simulink model "Clutchless_P2_Parallel"  (R2017b)
settings: Solver=FixedStepAuto  StartTime=0.0  StopTime=length(Speed)  FixedStep=0.01  MaxStep=0.01  RelTol=1e-3  EnableMultiTasking=on
PostLoadFcn:
  | , if any(exist('dsrtsu_mdlpostloadfcn', 'file') == [2, 3, 6]), try dsrtsu_mdlpostloadfcn('Execute', bdroot); catch fprintf('Error in PostLoadFcn (dsrtsu_mdlpostloadfcn) for model "%s":\n %s\n', bdroot, lasterr); end, end,
undefined symbols (not defined in the file): Actuators, APP1_OOR, APP2_OOR, APP_Mismatch, Brk_Flt, cal, Chassis, ClutchEngag, Clutchless_HSC, eng, Engine, EngineTorqueReal, EngOverTemp, ENGTRQ_MSMCH_Degraded_CP, ENGTRQ_MSMCH_ErrCritical_CP, ENGTRQ_MSMCH_LimpHome_CP, EngTrqMismatch, ess, ESSOverTemp, g, gb, Grade, KeyPos_Flt, lib_Actuators, lib_Chassis, lib_Clutchless_HSC, lib_EMachine_2017a, lib_Sensors_2017a, LossCAN, Machine, MCUOverTemp, mot, MotDirMismatch, motor_Trq, MotOverTemp, MotTrqMismatch, mph2ms, PRNDL_Flt, RegenFault, rho, Sensors, t_amb, time, tloop, veh, Vehicle
libraries: simulink x96, EC2_libraries x6, autolibmappedmotor x3, powerlib_meascontrol x2, CalculationGallon x1, lib_DCDC x1, lib_Differential x1, lib_HVESS x1, lib_Engine x1, lib_OBC x1, Scope_new x1, lib_Transmission x1
(part 2 of 10)

== system Clutchless_P2_Parallel/Camaro Plant Model/Scopes/AxlTrq_to_MtrTrq2 ==
  note: //From motor axle torque to motor torque//
  In1 : Inport
  Compare To Constant : simulink/Logic and Bit Operations/Compare To Constant  relop===  const=0  OutDataTypeStr=boolean
  Constant1 : Constant  Value=max(gb.plant.init.ratio.map)
  Constant5 : Constant  Value=fd.plant.init.ratio
  Divide : Product  Inputs=*//
  Rate Limiter : RateLimiter  RisingSlewLimit=mcu.plant.init.trq_uprate  FallingSlewLimit=mcu.plant.init.trq_derate
  Ratio Filter : Subsystem
  Switch : Switch  Criteria=u2 > Threshold
  Out1 : Outport
  wires:
  In1/1 -> Divide/1
  Constant5/1 -> Divide/2
  Divide/1 -> Rate Limiter/1
  [TransRatio] -> Ratio Filter/1(Ratio)
  Compare To Constant/1 -> Switch/2
  Constant1/1 -> Switch/1
  Rate Limiter/1 -> Out1/1
  Switch/1 -> Divide/3
  Ratio Filter/1(Filtered_Ratio) -> Switch/3, Compare To Constant/1

== system Clutchless_P2_Parallel/Clutchless_HSC/HSC/Camaro Fault Detection ==
  Sensors : Inport
  Component Diagnostic : Subsystem
  Input Conversions : Subsystem
  Signal Diagnostic : Subsystem
  SystemDiag : lib_SystemDiag/SystemDiag
  Diagnostic : Outport
  wires:
  Signal Diagnostic/1(SignalDiag) -> Component Diagnostic/1(SignalDiag)
  Component Diagnostic/1(CompDiag) -> SystemDiag/1
  Input Conversions/1(VehSig) -> Signal Diagnostic/1(VehSig)
  Sensors/1 -> Input Conversions/1(RawSig)
  SystemDiag/1 -> Diagnostic/1

== system Clutchless_P2_Parallel/Clutchless_HSC/HSC/Driver_Requests ==
  note: Driver management
  Sensors : Inport
  "Diagnostic " : Inport  Port=2
  "Controls " : Inport  Port=3
  APP_BPP to DrvIntndAxlTrq2 : Subsystem
  DriverRequests : Outport
  wires:
  "Controls "/1 -> APP_BPP to DrvIntndAxlTrq2/3(Controls)
  "Diagnostic "/1 -> APP_BPP to DrvIntndAxlTrq2/2(Diag)
  APP_BPP to DrvIntndAxlTrq2/1(IntndAxlTrq) -> DriverRequests/1
  Sensors/1 -> APP_BPP to DrvIntndAxlTrq2/1(Sensors)

== system Clutchless_P2_Parallel/Clutchless_HSC/HSC/Powertrain Manager ==
  Sensors : Inport
  Driver Request : Inport  Port=2
  Fault Detection : Inport  Port=3
  Ground : Ground
  HV Manager : Subsystem  AncestorBlock=lib_HVManager_PostIMG_2017a/HV Manager
  Output Conversion : Subsystem
  Thermal Manager : Subsystem  AncestorBlock=lib_ThermalManager/Thermal Manager
  Torque Distribution : Subsystem  AncestorBlock=lib_TorqueDistribution_2017a/Torque Distribution
  Out1 : Outport
  Controls : Outport  Port=2
  tag scope: HV_BUS_Status=global
  wires:
  Torque Distribution/1(Controls) -> HV Manager/2(Controls), Controls/1, [Controls]
  Ground/1 -> Output Conversion/9(In11)  "Trans_test"
  HV Manager/1(BMS_CAN) -> [BMS_CAN]
  HV Manager/2(HV_BUS_Status) -> [HV_BUS_Status]
  HV Manager/4(OBC_Digital) -> [OBC_Digital]
  HV Manager/3(OBC_CAN) -> [OBC_CAN]
  Driver Request/1 -> Torque Distribution/2(Driver Request)
  [BMS_CAN] -> Output Conversion/1(In1)  "BMS_CAN"
  [OBC_CAN] -> Output Conversion/2(In2)  "OBC_CAN"
  [MCU_CAN] -> Output Conversion/3(In3)  "MCU_CAN"
  [Controls] -> Output Conversion/4(In4)  "Controls"
  Output Conversion/1(Out1) -> Out1/1
  HV Manager/5(BMS_Digital) -> [BMS_Digital]
  [BMS_Digital] -> Output Conversion/5(In5)  "BMS_Digital"
  Fault Detection/1 -> Torque Distribution/3(Fault Detection)
  Thermal Manager/1(Out1) -> [Fuel_Pump_Control]
  HV Manager/6(Axiomatic_CAN) -> [Axiomatic_CAN]
  [Axiomatic_CAN] -> Output Conversion/8(In10)  "Axiomatic_CAN"
  [OBC_Digital] -> Output Conversion/7(In9)  "OBC_Digital"
  [Fuel_Pump_Control] -> Output Conversion/6(In8)  "Fuel_Pump_Control"
  Sensors/1 -> Thermal Manager/1(In2), HV Manager/1(Sensors), Torque Distribution/1(Sensors)

== system Clutchless_P2_Parallel/Fault Trigger /Component Diagnostics setting/Mismch type ==
  In1 : Inport
  Constant : Constant  Value=cal.ENGTRQ_MSMCH.Degraded_CP+1
  Constant1 : Constant  Value=cal.ENGTRQ_MSMCH.LimpHome_CP+1
  Constant2 : Constant  Value=cal.ENGTRQ_MSMCH.ErrCritical_CP+1
  Constant3 : Constant  Value=0
  Multiport Switch : MultiPortSwitch  DataPortOrder=Zero-based contiguous  Inputs=4
  Out1 : Outport
  wires:
  Constant1/1 -> Multiport Switch/4
  Constant2/1 -> Multiport Switch/5
  In1/1 -> Multiport Switch/1
  Multiport Switch/1 -> Out1/1
  Constant3/1 -> Multiport Switch/2
  Constant/1 -> Multiport Switch/3

== system Clutchless_P2_Parallel/Fault Trigger /Component Diagnostics setting/Mismch type1 ==
  In1 : Inport
  Constant : Constant  Value=cal.MOTTRQ_MSMCH.Degraded_CP+1
  Constant1 : Constant  Value=cal.MOTTRQ_MSMCH.LimpHome_CP+1
  Constant2 : Constant  Value=cal.ENGTRQ_MSMCH.ErrCritical_CP+1
  Constant3 : Constant  Value=0
  Multiport Switch : MultiPortSwitch  DataPortOrder=Zero-based contiguous  Inputs=4
  Out1 : Outport
  wires:
  Constant/1 -> Multiport Switch/3
  Constant3/1 -> Multiport Switch/2
  Multiport Switch/1 -> Out1/1
  In1/1 -> Multiport Switch/1
  Constant2/1 -> Multiport Switch/5
  Constant1/1 -> Multiport Switch/4

== system Clutchless_P2_Parallel/Fault Trigger /Component Diagnostics setting/Override  ClutchEngag ==
  note: Override Switch Subsystem
  note: This subsystem is used to override the model value of a signal to a constant value
  In1 : Inport
  Constant : Constant  Value=0
  Multiport Switch : MultiPortSwitch  DataPortOrder=Zero-based contiguous  Inputs=2
  Signal Override Switch 0 = Use Model 1 = Use Constant : Constant  Value=ClutchEngagFlt
  Out1 : Outport
  wires:
  Constant/1 -> Multiport Switch/3
  Multiport Switch/1 -> Out1/1
  In1/1 -> Multiport Switch/2
  Signal Override Switch 0 = Use Model 1 = Use Constant/1 -> Multiport Switch/1

== system Clutchless_P2_Parallel/Fault Trigger /Component Diagnostics setting/Override  ESSOverTemp ==
  note: This subsystem is used to override the model value of a signal to a constant value
  note: Override Switch Subsystem
  In1 : Inport
  Constant : Constant  Value=0
  Multiport Switch : MultiPortSwitch  DataPortOrder=Zero-based contiguous  Inputs=2
  Signal Override Switch 0 = Use Model 1 = Use Constant : Constant  Value=ESSOverTemp_ON
  Out1 : Outport
  wires:
  Signal Override Switch 0 = Use Model 1 = Use Constant/1 -> Multiport Switch/1
  In1/1 -> Multiport Switch/2
  Multiport Switch/1 -> Out1/1
  Constant/1 -> Multiport Switch/3

== system Clutchless_P2_Parallel/Fault Trigger /Component Diagnostics setting/Override  EngOverTemp ==
  note: Override Switch Subsystem
  note: This subsystem is used to override the model value of a signal to a constant value
  In1 : Inport
  Constant : Constant  Value=0
  Multiport Switch : MultiPortSwitch  DataPortOrder=Zero-based contiguous  Inputs=2
  Signal Override Switch 0 = Use Model 1 = Use Constant : Constant  Value=EngOverTemp_ON
  Out1 : Outport
  wires:
  Constant/1 -> Multiport Switch/3
  Multiport Switch/1 -> Out1/1
  In1/1 -> Multiport Switch/2
  Signal Override Switch 0 = Use Model 1 = Use Constant/1 -> Multiport Switch/1

== system Clutchless_P2_Parallel/Fault Trigger /Component Diagnostics setting/Override  EngTrqMismatch ==
  note: This subsystem is used to override the model value of a signal to a constant value
  note: Override Switch Subsystem
  In1 : Inport
  Constant : Constant  Value=0
  Multiport Switch : MultiPortSwitch  DataPortOrder=Zero-based contiguous  Inputs=2
  Signal Override Switch 0 = Use Model 1 = Use Constant : Constant  Value=EngTrqMismatch_ON
  Out1 : Outport
  wires:
  Signal Override Switch 0 = Use Model 1 = Use Constant/1 -> Multiport Switch/1
  In1/1 -> Multiport Switch/2
  Multiport Switch/1 -> Out1/1
  Constant/1 -> Multiport Switch/3

== system Clutchless_P2_Parallel/Fault Trigger /Component Diagnostics setting/Override  LossCAN ==
  note: Override Switch Subsystem
  note: This subsystem is used to override the model value of a signal to a constant value
  In1 : Inport
  Constant : Constant  Value=0
  Multiport Switch : MultiPortSwitch  DataPortOrder=Zero-based contiguous  Inputs=2
  Signal Override Switch 0 = Use Model 1 = Use Constant : Constant  Value=LossCAN_ON
  Out1 : Outport
  wires:
  Constant/1 -> Multiport Switch/3
  Multiport Switch/1 -> Out1/1
  In1/1 -> Multiport Switch/2
  Signal Override Switch 0 = Use Model 1 = Use Constant/1 -> Multiport Switch/1

== system Clutchless_P2_Parallel/Fault Trigger /Component Diagnostics setting/Override  MCUOverTemp ==
  note: This subsystem is used to override the model value of a signal to a constant value
  note: Override Switch Subsystem
  In1 : Inport
  Constant : Constant  Value=0
  Multiport Switch : MultiPortSwitch  DataPortOrder=Zero-based contiguous  Inputs=2
  Signal Override Switch 0 = Use Model 1 = Use Constant : Constant  Value=MCUOverTemp_ON
  Out1 : Outport
  wires:
  Signal Override Switch 0 = Use Model 1 = Use Constant/1 -> Multiport Switch/1
  In1/1 -> Multiport Switch/2
  Multiport Switch/1 -> Out1/1
  Constant/1 -> Multiport Switch/3

== system Clutchless_P2_Parallel/Fault Trigger /Component Diagnostics setting/Override  MotDirMismatch ==
  note: Override Switch Subsystem
  note: This subsystem is used to override the model value of a signal to a constant value
  In1 : Inport
  Constant : Constant  Value=0
  Multiport Switch : MultiPortSwitch  DataPortOrder=Zero-based contiguous  Inputs=2
  Signal Override Switch 0 = Use Model 1 = Use Constant : Constant  Value=MotDirMismatch_ON
  Out1 : Outport
  wires:
  Constant/1 -> Multiport Switch/3
  Multiport Switch/1 -> Out1/1
  In1/1 -> Multiport Switch/2
  Signal Override Switch 0 = Use Model 1 = Use Constant/1 -> Multiport Switch/1

== system Clutchless_P2_Parallel/Fault Trigger /Component Diagnostics setting/Override  MotOverTemp ==
  note: Override Switch Subsystem
  note: This subsystem is used to override the model value of a signal to a constant value
  In1 : Inport
  Constant : Constant  Value=0
  Multiport Switch : MultiPortSwitch  DataPortOrder=Zero-based contiguous  Inputs=2
  Signal Override Switch 0 = Use Model 1 = Use Constant : Constant  Value=MotOverTemp_ON
  Out1 : Outport
  wires:
  Constant/1 -> Multiport Switch/3
  Multiport Switch/1 -> Out1/1
  In1/1 -> Multiport Switch/2
  Signal Override Switch 0 = Use Model 1 = Use Constant/1 -> Multiport Switch/1

== system Clutchless_P2_Parallel/Fault Trigger /Component Diagnostics setting/Override  MotTrqMismatch ==
  note: This subsystem is used to override the model value of a signal to a constant value
  note: Override Switch Subsystem
  In1 : Inport
  Constant : Constant  Value=0
  Multiport Switch : MultiPortSwitch  DataPortOrder=Zero-based contiguous  Inputs=2
  Signal Override Switch 0 = Use Model 1 = Use Constant : Constant  Value=MotTrqMismatch_ON
  Out1 : Outport
  wires:
  Signal Override Switch 0 = Use Model 1 = Use Constant/1 -> Multiport Switch/1
  In1/1 -> Multiport Switch/2
  Multiport Switch/1 -> Out1/1
  Constant/1 -> Multiport Switch/3

== system Clutchless_P2_Parallel/Fault Trigger /Driver Interface Diagnostics setting/Override  APP1_OOR ==
  note: Signal Override Switch
      | 0 = Use Model
      | 1 = Use Constant
  note: Override Switch Subsystem
  note: This subsystem is used to override the model value of a signal to a constant value
  In1 : Inport
  APP1_OOR_ON : Constant  Value=APP1_OOR_ON
  Constant : Constant  Value=0
  Multiport Switch : MultiPortSwitch  DataPortOrder=Zero-based contiguous  Inputs=2
  Out1 : Outport
  wires:
  Constant/1 -> Multiport Switch/3
  Multiport Switch/1 -> Out1/1
  In1/1 -> Multiport Switch/2
  APP1_OOR_ON/1 -> Multiport Switch/1

== system Clutchless_P2_Parallel/Fault Trigger /Driver Interface Diagnostics setting/Override  APP2_OOR ==
  note: Signal Override Switch
      | 0 = Use Model
      | 1 = Use Constant
  note: This subsystem is used to override the model value of a signal to a constant value
  note: Override Switch Subsystem
  In1 : Inport
  APP2_OOR_ON : Constant  Value=APP2_OOR_ON
  Constant : Constant  Value=0
  Multiport Switch : MultiPortSwitch  DataPortOrder=Zero-based contiguous  Inputs=2
  Out1 : Outport
  wires:
  APP2_OOR_ON/1 -> Multiport Switch/1
  In1/1 -> Multiport Switch/2
  Multiport Switch/1 -> Out1/1
  Constant/1 -> Multiport Switch/3

== system Clutchless_P2_Parallel/Fault Trigger /Driver Interface Diagnostics setting/Override  APP_Mismatch ==
  note: Signal Override Switch
      | 0 = Use Model
      | 1 = Use Constant
  note: Override Switch Subsystem
  note: This subsystem is used to override the model value of a signal to a constant value
  In1 : Inport
  APP_Mismatch_Override : Constant  Value=Mismatch_APP_ON
  Constant : Constant  Value=0
  Multiport Switch : MultiPortSwitch  DataPortOrder=Zero-based contiguous  Inputs=2
  Out1 : Outport
  wires:
  Constant/1 -> Multiport Switch/3
  Multiport Switch/1 -> Out1/1
  In1/1 -> Multiport Switch/2
  APP_Mismatch_Override/1 -> Multiport Switch/1

== system Clutchless_P2_Parallel/Fault Trigger /Driver Interface Diagnostics setting/Override  BPP_Flt ==
  note: Signal Override Switch
      | 0 = Use Model
      | 1 = Use Constant
  note: This subsystem is used to override the model value of a signal to a constant value
  note: Override Switch Subsystem
  In1 : Inport
  Brk_Flt_ON : Constant  Value=Brk_Flt_ON
  Constant : Constant  Value=0
  Multiport Switch : MultiPortSwitch  DataPortOrder=Zero-based contiguous  Inputs=2
  Out1 : Outport
  wires:
  Brk_Flt_ON/1 -> Multiport Switch/1
  In1/1 -> Multiport Switch/2
  Multiport Switch/1 -> Out1/1
  Constant/1 -> Multiport Switch/3

== system Clutchless_P2_Parallel/Fault Trigger /Driver Interface Diagnostics setting/Override  KeyPos_Flt ==
  note: Signal Override Switch
      | 0 = Use Model
      | 1 = Use Constant
  note: Override Switch Subsystem
  note: This subsystem is used to override the model value of a signal to a constant value
  In1 : Inport
  Constant : Constant  Value=0
  KeyPos_Flt_ON : Constant  Value=KeyPos_Flt_ON
  Multiport Switch : MultiPortSwitch  DataPortOrder=Zero-based contiguous  Inputs=2
  Out1 : Outport
  wires:
  Constant/1 -> Multiport Switch/3
  Multiport Switch/1 -> Out1/1
  In1/1 -> Multiport Switch/2
  KeyPos_Flt_ON/1 -> Multiport Switch/1

== system Clutchless_P2_Parallel/Fault Trigger /Driver Interface Diagnostics setting/Override  PRNDL_Flt ==
  note: Signal Override Switch
      | 0 = Use Model
      | 1 = Use Constant
  note: This subsystem is used to override the model value of a signal to a constant value
  note: Override Switch Subsystem
  In1 : Inport
  Constant : Constant  Value=0
  Multiport Switch : MultiPortSwitch  DataPortOrder=Zero-based contiguous  Inputs=2
  PRNDL_Flt_ON : Constant  Value=PRNDL_Flt_ON
  Out1 : Outport
  wires:
  PRNDL_Flt_ON/1 -> Multiport Switch/1
  In1/1 -> Multiport Switch/2
  Multiport Switch/1 -> Out1/1
  Constant/1 -> Multiport Switch/3

== system Clutchless_P2_Parallel/Sensors/CAN/EBCAN ==
  In1 : Inport
  BMS_Antrieb : Subsystem
  Bus Creator : BusCreator  Inputs=3
  Bus Selector : BusSelector  OutputSignals=ECM_CAN,BMS_CAN.BMS_Hybrid
  CCM : Subsystem
  ECM : Subsystem
  Out1 : Outport
  wires:
  Bus Selector/2 -> CCM/1(In1), BMS_Antrieb/1(In1)  "<BMS_Hybrid>"
  Bus Selector/1 -> ECM/1(In1)  "<ECM_CAN>"
  In1/1 -> Bus Selector/1
  CCM/1(Out1) -> Bus Creator/3  "from_CCM"
  Bus Creator/1 -> Out1/1
  BMS_Antrieb/1(Out1) -> Bus Creator/2  "from_BMSAntrieb"
  ECM/1(Out1) -> Bus Creator/1  "from_ECM"

== system Clutchless_P2_Parallel/Sensors/CAN/HV_CAN ==
  In1 : Inport
  BMS_Hybrid : Subsystem
  Bus Creator : BusCreator  Inputs=3
  Bus Selector : BusSelector  OutputSignals=MCU_CAN,BMS_CAN.BMS_Plugin,OBC_CAN
  MCU : Subsystem
  OBC : Subsystem
  Out1 : Outport
  wires:
  Bus Selector/3 -> OBC/1(In1)  "<OBC_CAN>"
  Bus Selector/2 -> BMS_Hybrid/1(In1)  "<BMS_Plugin>"
  Bus Selector/1 -> MCU/1(In1)  "<MCU_CAN>"
  In1/1 -> Bus Selector/1
  Bus Creator/1 -> Out1/1
  OBC/1(Out1) -> Bus Creator/3  "from_OBC"
  BMS_Hybrid/1(Out1) -> Bus Creator/2  "from_BMSHybrid"
  MCU/1(Out1) -> Bus Creator/1  "from_MCU"

== system Clutchless_P2_Parallel/Sensors/CAN/VEH_CAN ==
  In1 : Inport
  BCM : Subsystem
  Bus Creator : BusCreator  Inputs=4
  Bus Selector : BusSelector  OutputSignals=TCM_CAN,BCM_CAN
  EBCM : Subsystem  Commented=on
  Ground : Ground  Commented=on
  Ground1 : Ground  Commented=on
  ICCM : Subsystem  Commented=on
  TCM : Subsystem
  Out1 : Outport
  wires:
  Ground/1 -> EBCM/1(In1)  "<EBCM>"
  Ground1/1 -> ICCM/1(In1)  "<ONSTAR>"
  Bus Selector/2 -> BCM/1(In1)  "<BCM_CAN>"
  Bus Selector/1 -> TCM/1(In1)  "<TCM_CAN>"
  Bus Creator/1 -> Out1/1
  EBCM/1(Out1) -> Bus Creator/4  "from_EBCM"
  ICCM/1(Out1) -> Bus Creator/3  "from_ICCM"
  BCM/1(Out1) -> Bus Creator/2  "from_BCM"
  TCM/1(Out1) -> Bus Creator/1  "from_TCM"
  In1/1 -> Bus Selector/1

== system Clutchless_P2_Parallel/Actuators/CAN/EBCAN/ISO_Hybrid_01_Req ==
  In1 : Inport
  Bus Creator : BusCreator  Inputs=1
  Bus Selector : BusSelector  OutputSignals=ISO_Hybrid_01_Req_Data_byte_3
  Data Type Conversion : DataTypeConversion
  Out1 : Outport
  wires:
  In1/1 -> Bus Selector/1
  Data Type Conversion/1 -> Bus Creator/1  "ISO_Hybrid_01_Req_Data_4"
  Bus Creator/1 -> Out1/1  "ISO_Hybrid_01_Req"
  Bus Selector/1 -> Data Type Conversion/1  "<ISO_Hybrid_01_Req_Data_byte_3>"

== system Clutchless_P2_Parallel/Actuators/CAN/EBCAN/PPEI_Platform_General_Status ==
  In1 : Inport
  Bus Creator : BusCreator  Inputs=1
  Data Type Conversion : DataTypeConversion
  Out1 : Outport
  wires:
  Bus Creator/1 -> Out1/1  "PPEI_Platform_General_Status"
  Data Type Conversion/1 -> Bus Creator/1  "SysPwrMd"
  In1/1 -> Data Type Conversion/1

== system Clutchless_P2_Parallel/Actuators/CAN/EBCAN/PPEI_Trans_General_Status_2 ==
  In1 : Inport
  Bus Creator : BusCreator  Inputs=1
  Data Type Conversion : DataTypeConversion
  Out1 : Outport
  wires:
  In1/1 -> Data Type Conversion/1
  Data Type Conversion/1 -> Bus Creator/1  "TrnsShftLvrPos"
  Bus Creator/1 -> Out1/1  "PPEI_Trans_General_Status_2"

== system Clutchless_P2_Parallel/Actuators/CAN/VEH_CAN/BCM ==
  In1 : Inport
  Bus Creator : BusCreator  Inputs=1
  Bus Selector : BusSelector  OutputSignals=Controls.powerMode
  Out1 : Outport
  wires:
  In1/1 -> Bus Selector/1
  Bus Selector/1 -> Bus Creator/1  "<powerMode>"
  Bus Creator/1 -> Out1/1

== system Clutchless_P2_Parallel/Actuators/CAN/VEH_CAN/EBCM ==
  In1 : Inport
  Out1 : Outport
  wires:
  In1/1 -> Out1/1

== system Clutchless_P2_Parallel/Actuators/CAN/VEH_CAN/ICCM ==
  In1 : Inport
  Out1 : Outport
  wires:
  In1/1 -> Out1/1

== system Clutchless_P2_Parallel/Camaro Plant Model/E-Machine/IMG Plant/ Actuators ==
  In1 : Inport
  Bus Selector : BusSelector  OutputSignals=MotTrqCmd,Direction_Command,InverterEnabled
  MotTrqCmd : Outport
  DirectionCommand : Outport  Port=2
  InverterEnabled : Outport  Port=3
  wires:
  In1/1 -> Bus Selector/1
  Bus Selector/1 -> MotTrqCmd/1  "<MotTrqCmd>"
  Bus Selector/2 -> DirectionCommand/1  "<Direction_Command>"
  Bus Selector/3 -> InverterEnabled/1  "<InverterEnabled>"

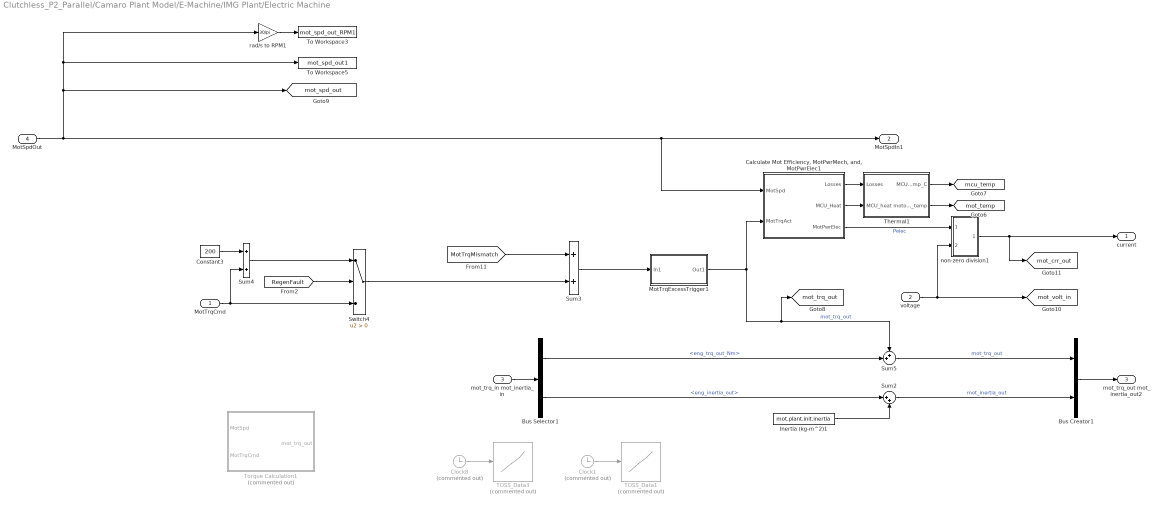
== system Clutchless_P2_Parallel/Camaro Plant Model/E-Machine/IMG Plant/Electric Machine ==
  MotTrqCmd : Inport
  voltage : Inport  Port=2
  mot_trq_in mot_inertia_in : Inport  Port=3
  MotSpdOut : Inport  Port=4
  Bus Creator1 : BusCreator  Inputs=2
  Bus Selector1 : BusSelector  OutputSignals=eng_trq_out_Nm,eng_inertia_out
  "Calculate Mot Efficiency, MotPwrMech, and, MotPwrElec1" : Subsystem
  Clock1 : Clock  Commented=on
  Clock8 : Clock  Commented=on
  Constant3 : Constant  Value=200
  Inertia (kg-m^2)1 : Constant  Value=mot.plant.init.inertia
  MotTrqExcessTrigger1 : Subsystem
  Sum2 : Sum  Inputs=|++
  Sum3 : Sum
  Sum4 : Sum
  Sum5 : Sum  Inputs=++|
  Switch4 : Switch  Criteria=u2 > Threshold
  TOSS_Data1 : Lookup_n-D  Commented=on  NumberOfTableDimensions=1  BreakpointsForDimension1=time  Table=EngineTorqueReal  InternalRulePriority=Speed  RndMeth=Simplest  InputSameDT=on
  TOSS_Data3 : Lookup_n-D  Commented=on  NumberOfTableDimensions=1  BreakpointsForDimension1=time  Table=motor_Trq  InternalRulePriority=Speed  RndMeth=Simplest  InputSameDT=on
  Thermal1 : Subsystem
  To Workspace3 : ToWorkspace  VariableName=mot_spd_out_RPM1  SampleTime=-1
      settings: Decimation=WORKSPACE_DECIMATION
  To Workspace5 : ToWorkspace  VariableName=mot_spd_out1  SampleTime=-1
      settings: Decimation=WORKSPACE_DECIMATION
  Torque Calculation1 : Subsystem  Commented=on
  non-zero division1 : Subsystem
      mask Display: disp('divider \n I1/I2')
  rad/s to RPM1 : Gain  Gain=30/pi
  current : Outport
  MotSpdIn1 : Outport  Port=2
  mot_trq_out mot_inertia_out2 : Outport  Port=3
  tag scope: mcu_temp=global, mot_crr_out=global, mot_spd_out=global, mot_temp=global, mot_trq_out=global, mot_volt_in=global
  wires:
  Thermal1/1(MCU_temp_C) -> [mcu_temp]
  Thermal1/2(motor_temp) -> [mot_temp]
  Constant3/1 -> Sum4/1
  [RegenFault] -> Switch4/2
  "Calculate Mot Efficiency, MotPwrMech, and, MotPwrElec1"/1(Losses) -> Thermal1/1(Losses)
  Sum4/1 -> Switch4/1
  Sum3/1 -> MotTrqExcessTrigger1/1(In1)
  "Calculate Mot Efficiency, MotPwrMech, and, MotPwrElec1"/2(MCU_Heat) -> Thermal1/2(MCU_heat)
  Switch4/1 -> Sum3/2
  "Calculate Mot Efficiency, MotPwrMech, and, MotPwrElec1"/3(MotPwrElec) -> non-zero division1/1(In1)  "Pelec"
  non-zero division1/1(Out1) -> [mot_crr_out], current/1
  MotTrqExcessTrigger1/1(Out1) -> [mot_trq_out], Sum5/1, "Calculate Mot Efficiency, MotPwrMech, and, MotPwrElec1"/2(MotTrqAct)  "mot_trq_out"
  MotTrqCmd/1 -> Sum4/2, Switch4/3
  voltage/1 -> non-zero division1/2(In2), [mot_volt_in]
  [MotTrqMismatch] -> Sum3/1
  Sum5/1 -> Bus Creator1/1  "mot_trq_out"
  Inertia (kg-m^2)1/1 -> Sum2/2
  Sum2/1 -> Bus Creator1/2  "mot_inertia_out"
  Bus Creator1/1 -> mot_trq_out mot_inertia_out2/1
  mot_trq_in mot_inertia_in/1 -> Bus Selector1/1
  Bus Selector1/2 -> Sum2/1  "<eng_inertia_out>"
  Bus Selector1/1 -> Sum5/2  "<eng_trq_out_Nm>"
  rad/s to RPM1/1 -> To Workspace3/1
  MotSpdOut/1 -> "Calculate Mot Efficiency, MotPwrMech, and, MotPwrElec1"/1(MotSpd), MotSpdIn1/1, [mot_spd_out], To Workspace5/1, rad/s to RPM1/1
  Clock8/1 -> TOSS_Data3/1
  Clock1/1 -> TOSS_Data1/1

== system Clutchless_P2_Parallel/Camaro Plant Model/E-Machine/IMG Plant/Sensors ==
  In2 : Inport
  In3 : Inport  Port=2
  In4 : Inport  Port=3
  In5 : Inport  Port=4
  In6 : Inport  Port=5
  In1 : Inport  Port=6
  In7 : Inport  Port=7
  Bus Creator : BusCreator  Inputs=7
  Out1 : Outport
  wires:
  Bus Creator/1 -> Out1/1
  In2/1 -> Bus Creator/1  "mot_spd_out"
  In4/1 -> Bus Creator/3  "mot_crr_out"
  In5/1 -> Bus Creator/4  "mot_volt_in"
  In3/1 -> Bus Creator/2  "mot_trq_out"
  In6/1 -> Bus Creator/5  "mot_temp"
  In1/1 -> Bus Creator/6  "mcu_temp"
  In7/1 -> Bus Creator/7  "clt_plant_spd_in"

== system Clutchless_P2_Parallel/Camaro Plant Model/E-Machine/IMG Plant2/ Actuators ==
  In1 : Inport
  Bus Selector : BusSelector  OutputSignals=MotTrqCmd,Direction_Command,InverterEnabled
  Out2 : Outport
  Out3 : Outport  Port=2
  Out4 : Outport  Port=3
  wires:
  Bus Selector/3 -> Out4/1  "<InverterEnabled>"
  Bus Selector/2 -> Out3/1  "<Direction_Command>"
  In1/1 -> Bus Selector/1
  Bus Selector/1 -> Out2/1  "<MotTrqCmd>"

== system Clutchless_P2_Parallel/Camaro Plant Model/E-Machine/IMG Plant2/Calculate Mot Efficiency, MotPwrMech, and, MotPwrElec ==
  note: Pelec_req = Pmech_req*Eff^k,
      | k = -1 if Trq >= 0,
      | k = 1 if Trq < 0
  MotSpd : Inport
  MotTrqAct : Inport  Port=2
  -1 : Gain  Gain=8
  "-1 when + 1 when - " : Gain  Gain=-1
  -2 : Gain  Gain=tloop
  2-D Lookup Table : Lookup_n-D  BreakpointsForDimension1=mot.plant.init.eff_trq.idx2_trq  BreakpointsForDimension2=mot.plant.init.eff_trq.idx1_spd  Table=mot.plant.init.eff_trq.map  InternalRulePriority=Speed  RndMeth=Simplest  InputSameDT=on
  Abs{,1..3} (4 alike) : Abs
  Add : Sum  Inputs=-+
  Add1 : Sum  Inputs=+-
  Add2 : Sum  Commented=on
  Constant : Constant  Value=1-0.8
  Constant1 : Constant  Commented=on  Value=mot.plant.init.mcu_mass
  Constant2 : Constant  Commented=on  Value=mot.plant.init.specific_heat
  Divide : Product  Commented=on  Inputs=*/
  Gain2 : Gain  Gain=1/100
  Lower Limit : Subsystem  Commented=on  mask{Lolimit=t_amb+20}
      mask prompts: Lolimit "Lower Limit"
  MCUOverTemp Fault : Subsystem  Commented=on
  MCU_WEGPmp : Constant  Value=0
  Math Function1 : Math  Operator=pow  SaturateOnIntegerOverflow=on
  Memory : Memory
  Memory1 : Memory  Commented=on
  Product : Product
  Product1 : Product
  Product2 : Product
  Product3 : Product  Commented=on
  Sign : Signum
  rad/s to rpm : Gain  Gain=30/pi
  Losses : Outport
  MotPwrElec : Outport  Port=2
  MCU_Heat : Outport  Port=3
  wires:
  Lower Limit/1(Out1) -> Memory1/1, MCUOverTemp Fault/1(In1)
  Add2/1 -> Lower Limit/1(In1)
  Memory1/1 -> Add2/2
  Divide/1 -> Add2/1
  Product3/1 -> Divide/2
  Constant2/1 -> Product3/2
  Constant1/1 -> Product3/1
  -2/1 -> MCU_Heat/1
  -1/1 -> Add1/2
  Add1/1 -> -2/1
  MCU_WEGPmp/1 -> -1/1
  Abs3/1 -> Add1/1
  Product2/1 -> Abs3/1
  Constant/1 -> Product2/2
  Memory/1 -> Sign/1
  Math Function1/1 -> Product1/2
  Add/1 -> Abs2/1
  Abs2/1 -> Losses/1
  "-1 when + 1 when - "/1 -> Math Function1/2
  MotSpd/1 -> rad/s to rpm/1, Product/2
  MotTrqAct/1 -> Abs/1, Product/1, Memory/1
  Product/1 -> Product1/1, Add/1  "MotPwrMech"
  Product1/1 -> MotPwrElec/1, Add/2, Product2/1  "MotPwrElec"
  2-D Lookup Table/1 -> Gain2/1
  Gain2/1 -> Math Function1/1
  Abs/1 -> 2-D Lookup Table/1
  Sign/1 -> "-1 when + 1 when - "/1
  Abs1/1 -> 2-D Lookup Table/2
  rad/s to rpm/1 -> Abs1/1

== system Clutchless_P2_Parallel/Camaro Plant Model/E-Machine/IMG Plant2/MotTrqExcessTrigger ==
  In1 : Inport
  Bias : Bias  Bias=55
  Bias1 : Bias  Bias=25
  Constant : Constant  Value=0
  Multiport Switch : MultiPortSwitch  DataPortOrder=Zero-based contiguous
  Out1 : Outport
  tag scope: MotTrqExcessTrig=global
  wires:
  Constant/1 -> Multiport Switch/1, [MotTrqExcessTrig]
  Bias1/1 -> Multiport Switch/3
  In1/1 -> Bias1/1, Bias/1, Multiport Switch/2
  Bias/1 -> Multiport Switch/4
  Multiport Switch/1 -> Out1/1

== system Clutchless_P2_Parallel/Camaro Plant Model/E-Machine/IMG Plant2/Motor_Plant ==
  Trq_cmd : Inport
  Batt_volt : Inport  Port=2
  Speed_rad/sec : Inport  Port=3
  Add : Sum
  Bus Creator : BusCreator  Inputs=5
  Efficiency Calcs : Subsystem
  Memory : Memory
  Random Number : RandomNumber  Mean=0.1  Variance=0.1  SampleTime=0.01
  rad/sec to rpm : Gain  Gain=60/(2*3.14)
  Mot_out : Outport
  wires:
  Efficiency Calcs/3(Elec_power_W) -> Bus Creator/5
  Efficiency Calcs/2(Mech_power_W) -> Bus Creator/4
  Efficiency Calcs/1(Mot_current) -> Bus Creator/3
  Batt_volt/1 -> Efficiency Calcs/3(Batt_volt)
  Trq_cmd/1 -> Add/1
  Bus Creator/1 -> Mot_out/1
  Memory/1 -> Efficiency Calcs/2(Torq_cmd_Nm), Bus Creator/1  "Mot_Trq_Nm"
  Random Number/1 -> Add/2
  rad/sec to rpm/1 -> Efficiency Calcs/1(Speed_rpm), Bus Creator/2  "Mot_spd_rpm"
  Speed_rad/sec/1 -> rad/sec to rpm/1
  Add/1 -> Memory/1

== system Clutchless_P2_Parallel/Camaro Plant Model/E-Machine/IMG Plant2/Sensors ==
  In2 : Inport
  In3 : Inport  Port=2
  In4 : Inport  Port=3
  In5 : Inport  Port=4
  In6 : Inport  Port=5
  In1 : Inport  Port=6
  In7 : Inport  Port=7
  Bus Creator : BusCreator  Inputs=7
  Out1 : Outport
  wires:
  In7/1 -> Bus Creator/7  "clt_plant_spd_in"
  In1/1 -> Bus Creator/6  "mcu_temp"
  Bus Creator/1 -> Out1/1
  In2/1 -> Bus Creator/1  "mot_spd_out"
  In4/1 -> Bus Creator/3  "mot_crr_out"
  In5/1 -> Bus Creator/4  "mot_volt_in"
  In3/1 -> Bus Creator/2  "mot_trq_out"
  In6/1 -> Bus Creator/5  "mot_temp"

== system Clutchless_P2_Parallel/Camaro Plant Model/E-Machine/IMG Plant2/Thermal ==
  Losses : Inport
  Motor Thermal : Subsystem
  mot_temp_C : Outport
  wires:
  Motor Thermal/1(Out1) -> mot_temp_C/1
  Losses/1 -> Motor Thermal/1(In1)  "[W]"

== system Clutchless_P2_Parallel/Camaro Plant Model/E-Machine/IMG Plant2/Thermal1 ==
  Losses : Inport
  MCU_heat : Inport  Port=2
  MotInv_loop : Subsystem
  Motor Thermal : Subsystem  Commented=on
  MCU_temp_C : Outport
  motor_temp : Outport  Port=2
  wires:
  MotInv_loop/2(Out2) -> motor_temp/1
  MotInv_loop/1(Out1) -> MCU_temp_C/1
  Losses/1 -> MotInv_loop/1(In1)  "[W]"
  MCU_heat/1 -> MotInv_loop/2(In2)

== system Clutchless_P2_Parallel/Camaro Plant Model/E-Machine/IMG Plant2/Torque Calculation ==
  MotSpd : Inport
  MotTrqCmd : Inport  Port=2
  Abs : Abs
  Abs1 : Abs
  MinMax : MinMax  Inputs=2
  Product : Product
  Sign : Signum
  electric machine filter : Subsystem
  "max torque " : Subsystem
  mot_trq_out : Outport
  wires:
  Product/1 -> electric machine filter/1(trq)
  MotTrqCmd/1 -> Abs/1, Sign/1, "max torque "/1(cmd)
  electric machine filter/1(filtered) -> mot_trq_out/1
  Abs1/1 -> MinMax/2
  Abs/1 -> MinMax/1
  MinMax/1 -> Product/2
  Sign/1 -> Product/1
  MotSpd/1 -> "max torque "/2(speed)
  "max torque "/1(max torque) -> Abs1/1

== system Clutchless_P2_Parallel/Camaro Plant Model/E-Machine/IMG Plant2/non-zero division ==
  note: and finally, the expression is: (u[1] \ u[2]) * 1 = u[1] \ u[2]
  note: (u[2]!=0) is true then returns 1
  note: if u[2] != 0, then output == u[1]\u[2]:
  note: (u[2]==0) is false then returns 0, thus (u[2]+(u[2]==0)) is equal to u[2]+0=u[2]
  note: and finally, the expression is: (u[1] \ 1) * 0 = 0
  note: (u[2]!=0) is false then returns 0
  note: if u[2] == 0, then output == 0:
  note: (u[2]==0) is true then returns 1, thus (u[2]+(u[2]==0)) is equal to 0+1=1
  note: original idea from Phil Sharer - ANL
      | original formula: u[1]\(u[2]+eps)*(u[2]!=0)
      | changes done by Gerald ZINI (dgey) - ANL (05\02\2001)
  In1 : Inport
  In2 : Inport  Port=2
  Fcn : Fcn  Expr=u[1]/(u[2]+(u[2]==0))*(u[2]!=0)
  Mux : Mux  Inputs=2
  Out1 : Outport
  wires:
  In2/1 -> Mux/2
  Fcn/1 -> Out1/1
  In1/1 -> Mux/1
  Mux/1 -> Fcn/1

== system Clutchless_P2_Parallel/Camaro Plant Model/E-Machine/Soft MCU/Subsystem ==
  MCU_RollingAliveCnt : Subsystem
  D3_Power_On_Timer : Outport
  wires:
  MCU_RollingAliveCnt/1(Out1) -> D3_Power_On_Timer/1  "D3_Power_On_Timer"

== system Clutchless_P2_Parallel/Camaro Plant Model/E-Machine/Soft MCU/Torque Calculation1 ==
  MotTrqReq : Inport
  MotSpd : Inport  Port=2
  MotTrqFdbck : Inport  Port=3
  Abs : Abs
  Abs1 : Abs
  MinMax : MinMax  Inputs=2
  Product : Product
  Sign : Signum
  "max torque " : Subsystem
  mot_trq_out : Outport
  wires:
  Product/1 -> mot_trq_out/1
  "max torque "/1(max torque) -> Abs1/1
  MotSpd/1 -> "max torque "/2(speed)
  MotTrqReq/1 -> "max torque "/1(Req), Sign/1, Abs/1
  Sign/1 -> Product/1
  MinMax/1 -> Product/2
  Abs/1 -> MinMax/1
  Abs1/1 -> MinMax/2
  MotTrqFdbck/1 -> "max torque "/3(torque)

== system Clutchless_P2_Parallel/Camaro Plant Model/E-Machine/Soft MCU/Torque Calculation2 ==
  MotTrqReq : Inport
  MotSpd : Inport  Port=2
  MotTrqFdbck : Inport  Port=3
  mot_temp : Inport  Port=4
  mcu_temp : Inport  Port=5
  mot_volt_in : Inport  Port=6
  1-D Lookup Table : Lookup_n-D  NumberOfTableDimensions=1  BreakpointsForDimension1=[0,12600,12700,12800,12900,13000]  Table=[1,1,0.75,0.5,0.25,0]  InternalRulePriority=Speed  RndMeth=Simplest  InputSameDT=on
  1-D Lookup Table1 : Lookup_n-D  NumberOfTableDimensions=1  BreakpointsForDimension1=[0,410,415,420,425,430]  Table=[1,1,0.75,0.5,0.25,0]  InternalRulePriority=Speed  RndMeth=Simplest  InputSameDT=on
  1-D Lookup Table2 : Lookup_n-D  Commented=on  NumberOfTableDimensions=1  BreakpointsForDimension1=[0,90,100]  Table=[1,1,0]  InternalRulePriority=Speed  RndMeth=Simplest  InputSameDT=on
  1-D Lookup Table3 : Lookup_n-D  NumberOfTableDimensions=1  BreakpointsForDimension1=[0,150,170]  Table=[1,1,0]  InternalRulePriority=Speed  RndMeth=Simplest  InputSameDT=on
  Abs : Abs
  Abs1 : Abs
  Constant : Constant
  MinMax : MinMax  Inputs=2
  Product : Product
  Product1 : Product  Inputs=5
  Sign : Signum
  Terminator1 : Terminator
  "max torque " : Subsystem
  rad/s to RPM1 : Gain  Gain=30/pi
  mot_trq_out : Outport
  wires:
  Product/1 -> Product1/5
  "max torque "/1(max torque) -> Abs1/1
  MotSpd/1 -> rad/s to RPM1/1, "max torque "/2(speed)
  MotTrqReq/1 -> "max torque "/1(Req), Sign/1, Abs/1
  Sign/1 -> Product/1
  MinMax/1 -> Product/2
  Abs/1 -> MinMax/1
  Abs1/1 -> MinMax/2
  MotTrqFdbck/1 -> "max torque "/3(torque)
  rad/s to RPM1/1 -> 1-D Lookup Table/1
  Product1/1 -> mot_trq_out/1
  1-D Lookup Table/1 -> Product1/4
  mot_volt_in/1 -> 1-D Lookup Table1/1
  1-D Lookup Table1/1 -> Product1/3
  mot_temp/1 -> 1-D Lookup Table3/1
  mcu_temp/1 -> Terminator1/1
  Constant/1 -> Product1/2
  1-D Lookup Table3/1 -> Product1/1
